simulink model "Simple_wanderer_external"  (R2013a)
settings: Solver=FixedStepDiscrete  StartTime=0.0  StopTime=20  FixedStep=.1  RelTol=1e-3
libraries: ariac x3
settings Model: Creator=fbanser  LastModifiedBy=reedh
settings DataIOCC: SaveFormat=StructureWithTime
settings OptimizationCC: OptimizeModelRefInitCode=on  LifeSpan=1
settings RTWCC: SystemTargetFile=Aria.tlc  TemplateMakefile=ert_default_tmf  Description=Aria Robot Target  RTWVerbose=off  ProcessScript=Aria_make_rtw_hook  CustomInclude="\"C:\\users\\fbanser\\desktop\\wolf\\Aria_STF\\Include\\\" \"C:\\users\\fbanser\\desktop\\wolf\\Aria_STF\\lib\\\""  CustomLibrary=ariac_vc10_i386.lib AriaVC10.lib
settings CodeAppCC: IgnoreCustomStorageClasses=off
settings STFCustomTargetCC: GenerateSampleERTMain=on  CombineOutputUpdateFcns=on  ERTCustomFileBanners=on  SupportContinuousTime=off  SupportNonInlinedSFcns=off  MATLABClassNameForMDSCustomization=Simulink.SoftwareTarget.ERTCustomization  SystemTargetFile=Aria.tlc
settings ERTTargetCC: TargetLibSuffix=.lib  ParMdlRefBuildCompliant=off  CompOptLevelCompliant=off  ConcurrentExecutionCompliant=off  ERTFirstTimeCompliant=off  ModelStepFunctionPrototypeControlCompliant=off  CPPClassGenCompliant=off  ExtMode=on  ExtModeMexArgs=10.10.10.11  ERTCustomFileTemplate=Aria_file_process.tlc

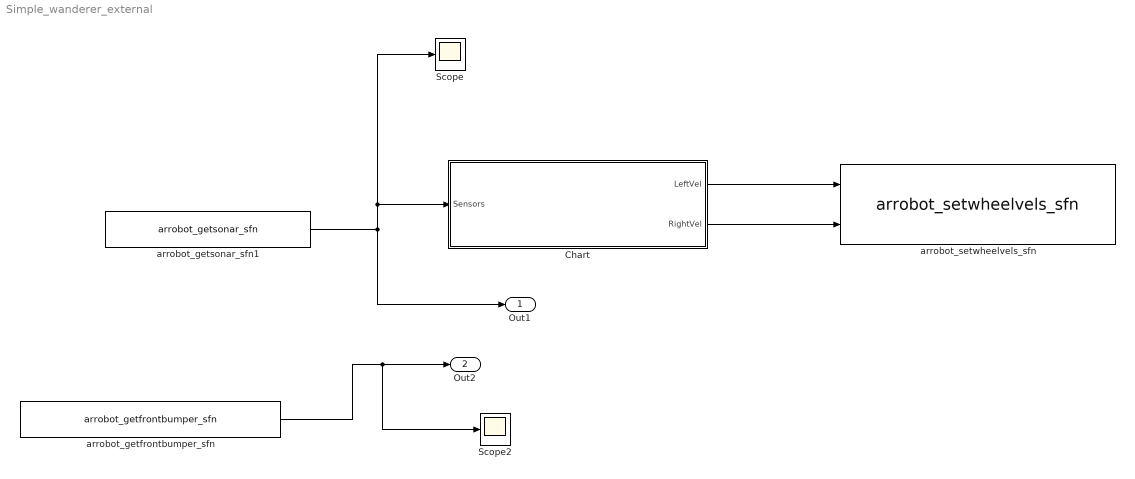
== system Simple_wanderer_external ==
  Chart : Stateflow chart  TreatAsAtomicUnit=on
  Scope : Scope
      settings: YMin=0  YMax=5000
  Scope2 : Scope
      settings: YMin=0  YMax=5000  SaveName=ScopeData2
  arrobot_getfrontbumper_sfn : ariac/arrobot_getfrontbumper_sfn  Description=Get range reading from one front bumper (0-indexed) of mobile robot  SFunctionSpec=int32 y1 = arrobot_get_front_bumper(int32 p1)  SParameter1=ones([1 1 ])  ShowSpec=on
      settings: AttributesFormatString=Get range reading from one front bumper (0-indexed) of mobile robot
  arrobot_getsonar_sfn1 : ariac/arrobot_getsonar_sfn  Description=Get range readings of all front sonar on mobile robot (mm)  SFunctionSpec=void arrobot_getsonar(double y1[16])  ShowSpec=on
      settings: AttributesFormatString=Get range readings of all front sonar on mobile robot (mm)
  arrobot_setwheelvels_sfn : ariac/arrobot_setwheelvels_sfn  Description=Set left, right wheel velocities separately (mm/sec), overrides vel, rotvel  SFunctionSpec=void arrobot_setwheelvels(double u1, double u2)  ShowSpec=on
      settings: AttributesFormatString=Set left, right wheel velocities separately (mm/sec), overrides vel, rotvel
  Out1 : Outport
  Out2 : Outport  Port=2
  wires:
  Chart/1(LeftVel) -> arrobot_setwheelvels_sfn/1
  Chart/2(RightVel) -> arrobot_setwheelvels_sfn/2
  arrobot_getsonar_sfn1/1 -> Scope/1, Chart/1(Sensors), Out1/1
  arrobot_getfrontbumper_sfn/1 -> Scope2/1, Out2/1

== stateflow chart Simple_wanderer_external/Chart ==
  state Modes [parallel]
    en,du:
    v0 = 60;
    settings: executionOrder=1
    state GoStraight
      en, du:
      RightVel = v0;
      LeftVel = v0;
    state Turn
      en:
      num = 0;
      state TurnL
        en:
        num=num+1;
        du :
        RightVel = v0;
        LeftVel = -v0;
      state TurnR
        en:
        num=num+1;
        du :
        RightVel = -v0;
        LeftVel = v0;
      (default) -> TurnR
      TurnL -> TurnR [order 1] : RIGHT
      TurnR -> TurnL [order 1] : LEFT
      TurnL -> (junction 209) [order 2]
      TurnR -> (junction 209) [order 2]
      (junction 209) -> (junction 212) : [num > 3]{send(Modes.LOCK)}
    state GoStraight1
      en, du:
      RightVel = v0;
      LeftVel = v0;
    (default) -> GoStraight
    Turn -> GoStraight [order 1] : FORWARD
    GoStraight -> Turn : TURN
    Turn -> GoStraight1 [order 2] : LOCK
    GoStraight1 -> Turn : after(20,TURN)
  state ObjectDetection [parallel]
    en,du:
    settings: executionOrder=2
    state logic
      en,du:
      (default) -> (junction 2) : {   i=1;
          |     detect_st =0;
          |     detect_end=0;}
      (junction 2) -> (junction 45) [order 1] : [i < 8]
      (junction 45) -> (junction 11)
      (junction 11) -> (junction 10) [order 1] : [Sensors[i]<200]
      (junction 10) -> (junction 26)
      (junction 11) -> (junction 16) [order 2]
      (junction 26) -> (junction 27) [order 1] : [detect_st == 0]
      (junction 26) -> (junction 32) [order 2] : {detect_end = i;}
      (junction 27) -> (junction 33) : {detect_st=i;
          | detect_end=i;}
      (junction 40) -> (junction 2) : {i = i + 1;}
      (junction 2) -> (junction 5) [order 2]
      (junction 33) -> (junction 32)
      (junction 32) -> (junction 14)
      (junction 14) -> (junction 16)
      (junction 16) -> (junction 40)
      (junction 5) -> (junction 41) [order 1] : [detect_st !=0]
          | {send(Modes.TURN)}
      (junction 5) -> (junction 43) [order 2] : {send(Modes.FORWARD)}
      (junction 41) -> (junction 195)
      (junction 195) -> (junction 192) [order 1] : [detect_st < 4]
      (junction 195) -> (junction 190) [order 2] : {send(Modes.LEFT)}
      (junction 192) -> (junction 193) : {send(Modes.RIGHT)}
      (junction 193) -> (junction 190)
      (junction 190) -> (junction 197) : //{send(Modes.TURN)}
    (default) -> logic
    logic -> logic
  data: i local double size=1; LeftVel output; RightVel output; Sensors input size=16; v0 local double size=1; detect_st local double size=1; detect_end local double size=1; num local double
  events: FORWARD local FUNCTION_CALL_EVENT; RIGHT local FUNCTION_CALL_EVENT; LEFT local FUNCTION_CALL_EVENT; TURN local FUNCTION_CALL_EVENT; LOCK local FUNCTION_CALL_EVENT
